simulink model "exercise_2"  (R2024b)
settings: Solver=VariableStepAuto  StartTime=0.0  StopTime=30  RelTol=1e-3
InitFcn:
  | disp('Loading EMG data...');
  | data = load('ES2_emg.mat');
  | 
  | signals = data.ES2_emg.signals; %30001x4
  | 
  | % Create time vector
  | Ts = 0.001;
  | 
  | num_samples = size(signals, 1);
  | 
  | time_vector = (0:num_samples-1)' * Ts;
  | 
  | raw_signals = [time_vector, signals];     % [Time, Data] 30001x5
  | 
  | disp('Data loaded and time vector created.');
undefined symbols (not defined in the file or in its folder): dspblkCoreblockFVToolHelper, gcbh
libraries: simulink x1, vrlib x1
settings Model: Creator=Lenovo  LastModifiedBy=philg
settings RTWCC: GPUComputeCapability=3.5

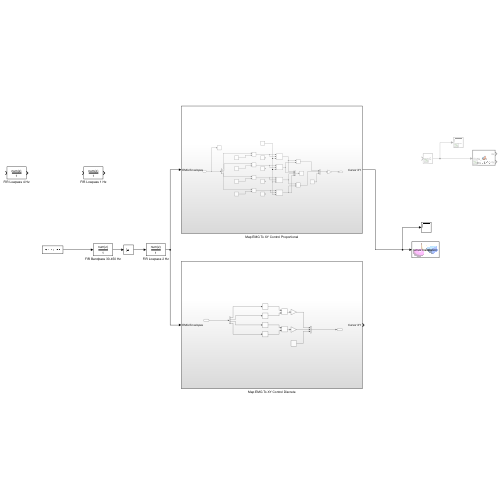
[thumbnail: Simulink's stored preview of the top-level diagram]
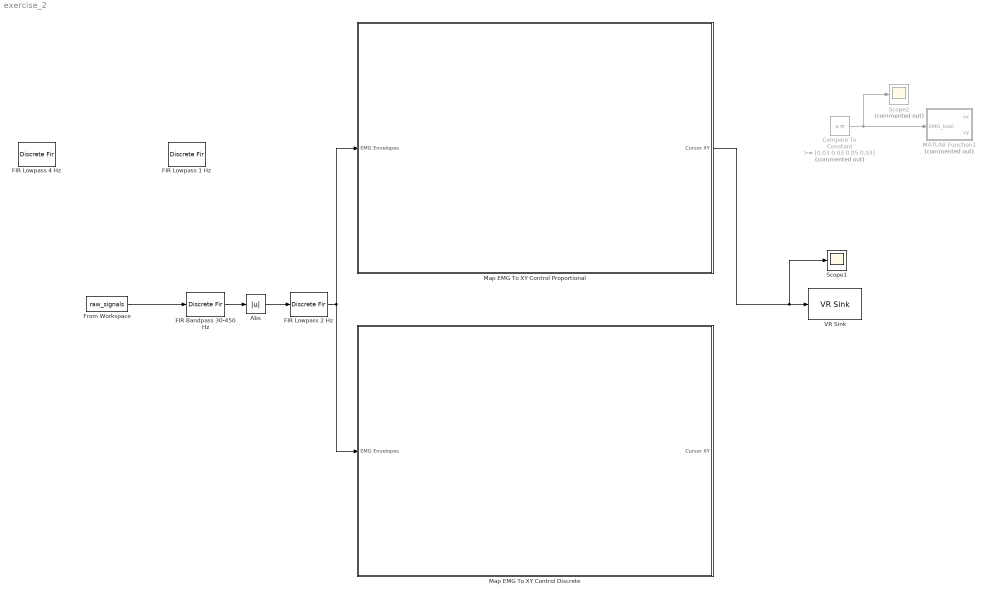
== system exercise_2 ==
  Abs : Abs  SaturateOnIntegerOverflow=off
  Compare To Constant : simulink/Logic and Bit Operations/Compare To Constant  Commented=on  relop=>=  const=[0.03 0.03 0.05 0.03]  OutDataTypeStr=boolean
  FIR Bandpass 30-450 Hz : DiscreteFir  LoadFcn=dspblkCoreblockFVToolHelper(gcbh,'load');  Coefficients="[-8.10293541537027e-19\t-3.13799520185598e-05\t0.000251238822487835\t-7.35585195773124e-05\t0.000453587009036026\t-5.48241954475755e-05\t0.000554039458485422\t4.97483585968486e-05\t0.000518298418947966\t0.000234825847688571\t0.000344868106957030\t0.000454492671302206\t7.42367722850010e-05\t0.000623668711562937\t-0.000215035260813460\t0.000638018355037721\t-0.000428411693080766\t0.000412323398702925\t-0.000492346253497723\t-7.32151941107620e-05\t-0.000392610326110226\t-0.000738389618732959\t-0.000194296309199899\t-0.00140147098700258\t-2.67755391451107e-05\t-0.00182292694473810\t-3.02446158704432e-05\t-0.00178800447531291\t-0.000279931546300458\t-0.00120105901039558\t-0.000720736999890264\t-0.000151617010484501\t-0.00114944281244077\t0.00108441997667148\t-0.00126812059408732\t0.00212315431164122\t-0.000803371308231205\t0.00261164270750469\t0.000347774958252984\t0.00237655862490170\t0.00200762616383089\t0.00151732924497948\t0.00370453799309888\t0.000391816859783294\t0.00478781780878167\t-0.000517393737049595\t0.00465103549158217\t-0.000815076420625186\t0.00299115819595611\t-0.000399035694710478\t5.46948140537493e-18\t0.000438159768149548\t-0.00360665955249822\t0.00107933853805041\t-0.00676512104325781\t0.000826820372932755\t-0.00840841141796561\t-0.000756472266055027\t-0.00786592790750236\t-0.00354486575800385\t-0.00516334155915873\t-0.00673247793132923\t-0.00108587616970502\t-0.00899406212038722\t0.00305387323693497\t-0.00891599399687903\t0.00588833338060455\t-0.00557304995218348\t0.00654480858629381\t0.000957532714956813\t0.00505467018427154\t0.00936565221898676\t0.00243032698697937\t0.0173076216385613\t0.000326908310342474\t0.0220367334307002\t0.000362615694512002\t0.0213007323886869\t0.00332041431143015\t0.0142164916289902\t0.00853414347158221\t0.00180077142969043\t0.0137346440678089\t-0.0130790555745118\t0.0154945444957208\t-0.0263888839979493\t0.0102044405590357\t-0.0340811239323958\t-0.00469104215828288\t-0.0333715334268134\t-0.0295953102570071\t-0.0237214188213651\t-0.0621935901464528\t-0.00717646729978686\t-0.0976680317641052\t0.0120910547504364\t-0.129701782916960\t0.0289309283941676\t-0.152019240052913\t0.0387140338197254\t0.840108126159796\t0.0387140338197254\t-0.152019240052913\t0.0289309283941676\t-0.129701782916960\t0.0120910547504364\t-0.0976680317641052\t-0.00717646729978686\t-0.0621935901464528\t-0.0237214188213651\t-0.0295953102570071\t-0.0333715334268134\t-0.00469104215828288\t-0.0340811239323958\t0.0102044405590357\t-0.0263888839979493\t0.0154945444957208\t-0.0130790555745118\t0.0137346440678089\t0.00180077142969043\t0.00853414347158221\t0.0142164916289902\t0.00332041431143015\t0.0213007323886869\t0.000362615694512002\t0.0220367334307002\t0.000326908310342474\t0.0173076216385613\t0.00243032698697937\t0.00936565221898676\t0.00505467018427154\t0.000957532714956813\t0.00654480858629381\t-0.00557304995218348\t0.00588833338060455\t-0.00891599399687903\t0.00305387323693497\t-0.00899406212038722\t-0.00108587616970502\t-0.00673247793132923\t-0.00516334155915873\t-0.00354486575800385\t-0.00786592790750236\t-0.000756472266055027\t-0.00840841141796561\t0.000826820372932755\t-0.00676512104325781\t0.00107933853805041\t-0.00360665955249822\t0.000438159768149548\t5.46948140537493e-18\t-0.000399035694710478\t0.00299115819595611\t-0.000815076420625186\t0.00465103549158217\t-0.000517393737049595\t0.00478781780878167\t0.000391816859783294\t0.00370453799309888\t0.00151732924497948\t0.00200762616383089\t0.00237655862490170\t0.000347774958252984\t0.00261164270750469\t-0.000803371308231205\t0.00212315431164122\t-0.00126812059408732\t0.00108441997667148\t-0.00114944281244077\t-0.000151617010484501\t-0.000720736999890264\t-0.00120105901039558\t-0.000279931546300458\t-0.00178800447531291\t-3.02446158704432e-05\t-0.00182292694473810\t-2.67755391451107e-05\t-0.00140147098700258\t-0.000194296309199899\t-0.000738389618732959\t-0.000392610326110226\t-7.32151941107620e-05\t-0.000492346253497723\t0.000412323398702925\t-0.000428411693080766\t0.000638018355037721\t-0.000215035260813460\t0.000623668711562937\t7.42367722850010e-05\t0.000454492671302206\t0.000344868106957030\t0.000234825847688571\t0.000518298418947966\t4.97483585968486e-05\t0.000554039458485422\t-5.48241954475755e-05\t0.000453587009036026\t-7.35585195773124e-05\t0.000251238822487835\t-3.13799520185598e-05\t-8.10293541537027e-19]"
      settings: CopyFcn=dspblkCoreblockFVToolHelper(gcbh,'copy');  DeleteFcn=dspblkCoreblockFVToolHelper(gcbh,'close');  ModelCloseFcn=dspblkCoreblockFVToolHelper(gcbh,'close');  PreSaveFcn=dspblkCoreblockFVToolHelper(gcbh,'presave');  PostSaveFcn=dspblkCoreblockFVToolHelper(gcbh,'postsave');  CloseFcn=dspblkCoreblockFVToolHelper(gcbh,'close');
  FIR Lowpass 1 Hz : DiscreteFir  LoadFcn=dspblkCoreblockFVToolHelper(gcbh,'load');  Coefficients="[0.00145895552195016\t0.00147647699724904\t0.00152708589850175\t0.00161064788035591\t0.00172689557077838\t0.00187542948856966\t0.00205571949944736\t0.00226710680535874\t0.00250880645948027\t0.00277991039718900\t0.00307939097115524\t0.00340610497661783\t0.00375879815087067\t0.00413611012902051\t0.00453657983618024\t0.00495865129444599\t0.00540067982127891\t0.00586093859427998\t0.00633762555581635\t0.00682887062953581\t0.00733274321949942\t0.00784725996147538\t0.00837039269487602\t0.00890007662288755\t0.00943421862754457\t0.00997070570584002\t0.0105074134924402\t0.0110422148341961\t0.0115729883814059\t0.0120976271606959\t0.0126140470944399\t0.0131201954318383\t0.0136140590571252\t0.0140936726408566\t0.0145571266008650\t0.0150025748402316\t0.0154282422305320\t0.0158324318096455\t0.0162135316645810\t0.0165700214710582\t0.0169004786629850\t0.0172035842064857\t0.0174781279547564\t0.0177230135617392\t0.0179372629344190\t0.0181200202054399\t0.0182705552097062\t0.0183882664506734\t0.0184726835441306\t0.0185234691294226\t0.0185404202402520\t0.0185234691294226\t0.0184726835441306\t0.0183882664506734\t0.0182705552097062\t0.0181200202054399\t0.0179372629344190\t0.0177230135617392\t0.0174781279547564\t0.0172035842064857\t0.0169004786629850\t0.0165700214710582\t0.0162135316645810\t0.0158324318096455\t0.0154282422305320\t0.0150025748402316\t0.0145571266008650\t0.0140936726408566\t0.0136140590571252\t0.0131201954318383\t0.0126140470944399\t0.0120976271606959\t0.0115729883814059\t0.0110422148341961\t0.0105074134924402\t0.00997070570584002\t0.00943421862754457\t0.00890007662288755\t0.00837039269487602\t0.00784725996147538\t0.00733274321949942\t0.00682887062953581\t0.00633762555581635\t0.00586093859427998\t0.00540067982127891\t0.00495865129444599\t0.00453657983618024\t0.00413611012902051\t0.00375879815087067\t0.00340610497661783\t0.00307939097115524\t0.00277991039718900\t0.00250880645948027\t0.00226710680535874\t0.00205571949944736\t0.00187542948856966\t0.00172689557077838\t0.00161064788035591\t0.00152708589850175\t0.00147647699724904\t0.00145895552195016]"
      settings: CopyFcn=dspblkCoreblockFVToolHelper(gcbh,'copy');  DeleteFcn=dspblkCoreblockFVToolHelper(gcbh,'close');  ModelCloseFcn=dspblkCoreblockFVToolHelper(gcbh,'close');  PreSaveFcn=dspblkCoreblockFVToolHelper(gcbh,'presave');  PostSaveFcn=dspblkCoreblockFVToolHelper(gcbh,'postsave');  CloseFcn=dspblkCoreblockFVToolHelper(gcbh,'close');
  FIR Lowpass 2 Hz : DiscreteFir  LoadFcn=dspblkCoreblockFVToolHelper(gcbh,'load');  Coefficients="[0.00139864560393775\t0.00141830449231384\t0.00146982131648521\t0.00155324926628869\t0.00166850446151114\t0.00181536567959752\t0.00199347469243198\t0.00220233721302816\t0.00244132445015437\t0.00270967526611006\t0.00300649893007320\t0.00333077845666962\t0.00368137451668602\t0.00405702990417315\t0.00445637454157589\t0.00487793100199644\t0.00532012052525699\t0.00578126950209092\t0.00625961639856882\t0.00675331909076696\t0.00726046257772301\t0.00777906703890488\t0.00830709620075384\t0.00884246597535979\t0.00938305333299221\t0.00992670536905287\t0.0104712485250389\t0.0110144979223157\t0.0115542667668999\t0.0120883757830458\t0.0126146626332217\t0.0131309912820480\t0.0136352612619558\t0.0141254167987079\t0.0145994557555005\t0.0150554383551358\t0.0154914956407191\t0.0159058376364745\t0.0162967611716058\t0.0166626573316245\t0.0170020185032373\t0.0173134449807100\t0.0175956511036037\t0.0178474708978982\t0.0180678631947665\t0.0182559162036399\t0.0184108515186824\t0.0185320275403735\t0.0186189422965697\t0.0186712356501485\t0.0186886908831464\t0.0186712356501485\t0.0186189422965697\t0.0185320275403735\t0.0184108515186824\t0.0182559162036399\t0.0180678631947665\t0.0178474708978982\t0.0175956511036037\t0.0173134449807100\t0.0170020185032373\t0.0166626573316245\t0.0162967611716058\t0.0159058376364745\t0.0154914956407191\t0.0150554383551358\t0.0145994557555005\t0.0141254167987079\t0.0136352612619558\t0.0131309912820480\t0.0126146626332217\t0.0120883757830458\t0.0115542667668999\t0.0110144979223157\t0.0104712485250389\t0.00992670536905287\t0.00938305333299221\t0.00884246597535979\t0.00830709620075384\t0.00777906703890488\t0.00726046257772301\t0.00675331909076696\t0.00625961639856882\t0.00578126950209092\t0.00532012052525699\t0.00487793100199644\t0.00445637454157589\t0.00405702990417315\t0.00368137451668602\t0.00333077845666962\t0.00300649893007320\t0.00270967526611006\t0.00244132445015437\t0.00220233721302816\t0.00199347469243198\t0.00181536567959752\t0.00166850446151114\t0.00155324926628869\t0.00146982131648521\t0.00141830449231384\t0.00139864560393775]"
      settings: CopyFcn=dspblkCoreblockFVToolHelper(gcbh,'copy');  DeleteFcn=dspblkCoreblockFVToolHelper(gcbh,'close');  ModelCloseFcn=dspblkCoreblockFVToolHelper(gcbh,'close');  PreSaveFcn=dspblkCoreblockFVToolHelper(gcbh,'presave');  PostSaveFcn=dspblkCoreblockFVToolHelper(gcbh,'postsave');  CloseFcn=dspblkCoreblockFVToolHelper(gcbh,'close');
  FIR Lowpass 4 Hz : DiscreteFir  LoadFcn=dspblkCoreblockFVToolHelper(gcbh,'load');  Coefficients=|
      | [0.00116777644563818	0.00119490819291279	0.00124922227014320	0.00133145140920837	0.00144218545141239	0.00158186587046618	0.00175078111120132	0.00194906277966055	0.00217668271516792	0.00243345096971649	0.00271901471455381	0.00303285808823172	0.00337430299465021	0.00374251085380398	0.00413648530206974	0.00455507583299189	0.00499698236366962	0.00546076070605930	0.00594482891681842	0.00644747449376846	0.00696686238168073	0.00750104374492508	0.00804796545960226	0.00860548027313650	0.00917135757496878	0.00974329471799020	0.0103189288267159	0.0108958490249486	0.0114716090128371	0.0120437399208192	0.0126097633659700	0.0131672046347607	0.0137136059151921	0.0142465395007019	0.0147636208881563	0.0152625216926406	0.0157409823026407	0.0161968242005666	0.0166279618753989	0.0170324142565235	0.0174083156005531	0.0177539257660950	0.0180676398149942	0.0183479968825372	0.0185936882634228	0.0188035646649597	0.0189766425839127	0.0191121097686568	0.0192093297337761	0.0192678452999316	0.0192873811376819	0.0192678452999316	0.0192093297337761	0.0191121097686568	0.0189766425839127	0.0188035646649597	0.0185936882634228	0.0183479968825372	0.0180676398149942	0.0177539257660950	0.0174083156005531	0.0170324142565235	0.0166279618753989	0.0161968242005666	0.0157409823026407	0.0152625216926406	0.0147636208881563	0.0142465395007019	0.0137136059151921	0.0131672046347607	0.0126097633659700	0.0120437399208192	0.0114716090128371	0.0108958490249486	0.0103189288267159	0.00974329471799020	0.00917135757496878	0.00860548027313650	0.00804796545960226	0.00750104374492508	0.00696686238168073	0.00644747449376846	0.00594482891681842	0.00546076070605930	0.00499698236366962	0.00455507583299189	0.00413648530206974	0.00374251085380398	0.00337430299465021	0.00303285808823172	0.00271901471455381	0.00243345096971649	0.00217668271516792	0.00194906277966055	0.00175078111120132	0.00158186587046618	0.00144218545141239	0.00133145140920837	0.00124922227014320	0.00119490819291279	0.00116777644563818
      |  ]
      settings: CopyFcn=dspblkCoreblockFVToolHelper(gcbh,'copy');  DeleteFcn=dspblkCoreblockFVToolHelper(gcbh,'close');  ModelCloseFcn=dspblkCoreblockFVToolHelper(gcbh,'close');  PreSaveFcn=dspblkCoreblockFVToolHelper(gcbh,'presave');  PostSaveFcn=dspblkCoreblockFVToolHelper(gcbh,'postsave');  CloseFcn=dspblkCoreblockFVToolHelper(gcbh,'close');
  From Workspace : FromWorkspace  VariableName=raw_signals  SampleTime=0.001  Interpolate=off  ZeroCross=off  OutputAfterFinalValue=Holding final value
  MATLAB Function1 : MATLAB Function  Commented=on  TreatAsAtomicUnit=on
  Map EMG To XY Control Discrete : Subsystem
  Map EMG To XY Control Proportional : Subsystem
  Scope1 : Scope
  Scope2 : Scope  Commented=on
  VR Sink : vrlib/VR Sink  InstantiateOnLoad=on  SampleTime=0.1  ViewEnable=on  RemoteChange=off  RemoteView=off  FieldsWritten=cursor.translation.3.1.1.double  WorldFileName=8_palline_color.wrl  AutoView=off  VideoDimensions=[]  AllowVariableSize=off
  wires:
  Abs/1 -> FIR Lowpass 2 Hz/1
  FIR Bandpass 30-450 Hz/1 -> Abs/1
  Compare To Constant/1 -> Scope2/1, MATLAB Function1/1(EMG_bool)
  From Workspace/1 -> FIR Bandpass 30-450 Hz/1
  FIR Lowpass 2 Hz/1 -> Map EMG To XY Control Proportional/1(EMG Envelopes), Map EMG To XY Control Discrete/1(EMG Envelopes)
  Map EMG To XY Control Proportional/1(Cursor XY) -> VR Sink/1, Scope1/1

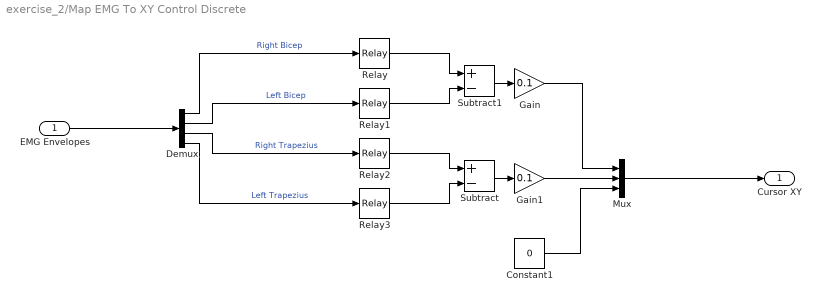
== system exercise_2/Map EMG To XY Control Discrete ==
  EMG Envelopes : Inport
  Constant1 : Constant  Value=0
  Demux : Demux
  Gain : Gain  Gain=0.1
  Gain1 : Gain  Gain=0.1
  Mux : Mux  Inputs=3
  Relay{,1..3} (4 alike) : Relay  OnSwitchValue=0.05  OffSwitchValue=0.03
  Subtract : Sum  Inputs=+-
  Subtract1 : Sum  Inputs=+-
  Cursor XY : Outport
  wires:
  Relay2/1 -> Subtract/1
  Relay/1 -> Subtract1/1
  Gain/1 -> Mux/1
  Constant1/1 -> Mux/3
  Demux/3 -> Relay2/1  "Right Trapezius"
  Demux/2 -> Relay1/1  "Left Bicep"
  Relay3/1 -> Subtract/2
  Demux/4 -> Relay3/1  "Left Trapezius"
  Demux/1 -> Relay/1  "Right Bicep"
  Relay1/1 -> Subtract1/2
  Subtract1/1 -> Gain/1
  Subtract/1 -> Gain1/1
  Gain1/1 -> Mux/2
  EMG Envelopes/1 -> Demux/1
  Mux/1 -> Cursor XY/1

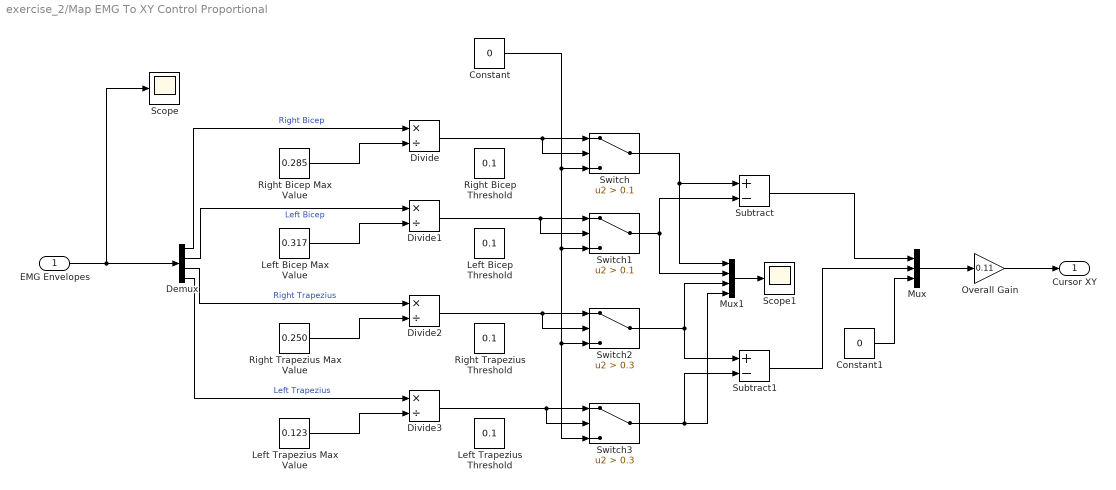
== system exercise_2/Map EMG To XY Control Proportional ==
  EMG Envelopes : Inport
  Constant : Constant  Value=0
  Constant1 : Constant  Value=0
  Demux : Demux
  Divide{,1..3} (4 alike) : Product  Inputs=*/
  Left Bicep Max Value : Constant  Value=0.317
  Left Bicep Threshold : Constant  Value=0.1
  Left Trapezius Max Value : Constant  Value=0.123
  Left Trapezius Threshold : Constant  Value=0.1
  Mux : Mux  Inputs=3
  Mux1 : Mux
  Overall Gain : Gain  Gain=0.11
  Right Bicep Max Value : Constant  Value=0.285
  Right Bicep Threshold : Constant  Value=0.1
  Right Trapezius Max Value : Constant  Value=0.250
  Right Trapezius Threshold : Constant  Value=0.1
  Scope : Scope
  Scope1 : Scope
  Subtract : Sum  Inputs=+-
  Subtract1 : Sum  Inputs=+-
  Switch : Switch  Criteria=u2 > Threshold  Threshold=0.1  SaturateOnIntegerOverflow=off  InputSameDT=off
  Switch1 : Switch  Criteria=u2 > Threshold  Threshold=0.1  SaturateOnIntegerOverflow=off  InputSameDT=off
  Switch2 : Switch  Criteria=u2 > Threshold  Threshold=0.3  SaturateOnIntegerOverflow=off  InputSameDT=off
  Switch3 : Switch  Criteria=u2 > Threshold  Threshold=0.3  SaturateOnIntegerOverflow=off  InputSameDT=off
  Cursor XY : Outport
  wires:
  Constant1/1 -> Mux/3
  Demux/3 -> Divide2/1  "Right Trapezius"
  Demux/2 -> Divide1/1  "Left Bicep"
  Demux/4 -> Divide3/1  "Left Trapezius"
  Demux/1 -> Divide/1  "Right Bicep"
  EMG Envelopes/1 -> Scope/1, Demux/1
  Right Bicep Max Value/1 -> Divide/2
  Left Bicep Max Value/1 -> Divide1/2
  Right Trapezius Max Value/1 -> Divide2/2
  Left Trapezius Max Value/1 -> Divide3/2
  Mux/1 -> Overall Gain/1
  Overall Gain/1 -> Cursor XY/1
  Constant/1 -> Switch3/3, Switch2/3, Switch1/3, Switch/3
  Divide/1 -> Switch/2, Switch/1
  Divide1/1 -> Switch1/2, Switch1/1
  Divide2/1 -> Switch2/2, Switch2/1
  Divide3/1 -> Switch3/2, Switch3/1
  Switch/1 -> Subtract/1, Mux1/1
  Switch1/1 -> Subtract/2, Mux1/2
  Switch2/1 -> Subtract1/1, Mux1/3
  Switch3/1 -> Subtract1/2, Mux1/4
  Mux1/1 -> Scope1/1
  Subtract/1 -> Mux/1
  Subtract1/1 -> Mux/2

== matlab function exercise_2/MATLAB Function1 ==
  data: EMG_bool input; vx output; vy output
function [vx, vy] = mapEMG(EMG_bool)
% EMG_bool è un vettore [1x4] di 0 o 1
% ch1: up, ch2: down, ch3: left, ch4: right

vx = 0;
vy = 0;

if EMG_bool(1)
    vy =  1; % up
end
if EMG_bool(2)
    vy = -1; % down
end
if EMG_bool(3)
    vx = -1; % left
end
if EMG_bool(4)
    vx =  1; % right
end
end
